simulink model "LagLead_With_saturation"  (Simulink 8.9)
settings: Solver=VariableStepAuto  StartTime=0.0  StopTime=10000  RelTol=1e-3
settings Model: Creator=maurice waked  LastModifiedBy=maurice waked
settings DataIOCC: LimitDataPoints=off  SaveFormat=Dataset  SignalLoggingSaveFormat=Dataset  ReturnWorkspaceOutputs=on
settings OptimizationCC: LifeSpan=auto
settings DebuggingCC: UnderspecifiedInitializationDetection=Simplified  MergeDetectMultiDrivingBlocksExec=error  FcnCallInpInsideContextMsg=error  StateNameClashWarn=none  SFUnexpectedBacktrackingDiag=error  SFNoUnconditionalDefaultTransitionDiag=error  SFExecutionAtInitializationDiag=warning
settings HardwareCC: ProdBitPerPointer=64  ProdBitPerSizeT=64  ProdBitPerPtrDiffT=64  ProdLargestAtomicFloat=Float  ProdIntDivRoundTo=Zero  ProdEndianess=LittleEndian  ProdWordSize=64  ProdHWDeviceType=Intel->x86-64 (Windows64)
settings ModelReferenceCC: PropagateSignalLabelsOutOfModel=on
settings SFSimCC: SimUseLocalCustomCode=on
settings RTWCC: RTWUseLocalCustomCode=on
settings GRTTargetCC: TargetLangStandard=C99 (ISO)  CombineOutputUpdateFcns=on  GRTInterface=off
settings ConfigComp: CovMetricSettings=dwe  CovHtmlReporting=off  CovSaveCumulativeToWorkspaceVar=off  CovSaveSingleToWorkspaceVar=off  CovExternalEMLEnable=on

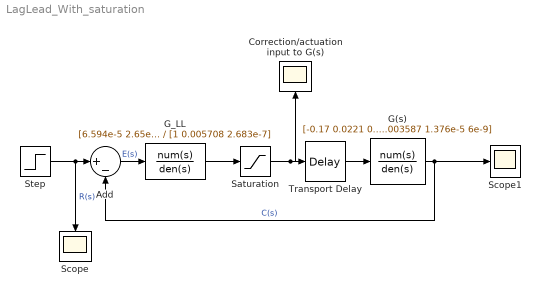
== system LagLead_With_saturation ==
  Add : Sum  Inputs=|+-
  Correction/actuation input to G(s) : Scope
  G(s) : TransferFcn  Numerator=[-0.17 0.0221 0.00068]  Denominator=[1 0.1345 0.003587 1.376e-5 6e-9]
  G_LL : TransferFcn  Numerator=[6.594e-5 2.65e-7 1.16e-10]  Denominator=[1 0.005708 2.683e-7]
  Saturation : Saturate  UpperLimit=2e-5  LowerLimit=0
  Scope : Scope
  Scope1 : Scope
  Step : Step  SampleTime=0
  Transport Delay : TransportDelay  DelayTime=8.5
  wires:
  Step/1 -> Scope/1, Add/1  "R(s)"
  Add/1 -> G_LL/1  "E(s)"
  G(s)/1 -> Scope1/1, Add/2  "C(s)"
  G_LL/1 -> Saturation/1
  Saturation/1 -> Transport Delay/1, Correction/actuation input to G(s)/1
  Transport Delay/1 -> G(s)/1
